simulink model "Model_14Bus_AC_DC_Microgrid"  (R2025a)
settings: Solver=ode23tb  StartTime=0.0  StopTime=0.1  MaxStep=1e-2  RelTol=1e-3
InitFcn:
  | Set_parameters_R2018
StopFcn:
  | Save_Data;
  | Graphics;
undefined symbols (not defined in the file): Clink, D1, Delta, dis1, dis10, dis11, dis12, dis13, dis14, dis2, dis3, dis4, dis5, dis6, dis7, dis8, dis9, Fc, Fnom, Hydride, Increment_MPPT, Ion, Ki_Ireg, Ki_VDCreg, Kp_Ireg, Kp_VDCreg, LimitL_Ireg, LimitL_VDCreg, Limits_MPPT, LimitU_Ireg, LimitU_VDCreg, Lithium, max_min, Metal, Nickel, P_Load_2, P_Load_3, Pnom, Pnom_T1, Pnom_T2, Pnom_T3, Pnom_xfo, Ql_Load_2, Ql_Load_3, R_Load_9, R_Load_DC, RL, Rl, RLff, Rls, sigbuilder_block, Ts, Ts_Control, Ts_Power, V1_LL_T3, Vf, Vfd, Vnom_dc, Vnom_DC, Vnom_Diesel ... (+5)
libraries: spsRMSLib x87, spsCurrentMeasurementLib x47, spsThreePhaseVIMeasurementLib x23, spsVoltageMeasurementLib x21, spsPowerLib x21, spsTHDLib x20, spsThreePhaseSeriesRLCBranchLib x20, spsSeriesRLCBranchLib x19, spsIGBTDiodeLib x14, spsThreePhaseBreakerLib x14, powerlib_extras x14, simulink x12
(part 1 of 9)
settings Model: Creator=Leony  LastModifiedBy=Sanny
settings SolverCC: ZeroCrossAlgorithm=Adaptive  AlgebraicLoopSolver=TrustRegion  SolverResetMethod=Robust
settings DataIOCC: LimitDataPoints=on  SaveFormat=Array  ReturnWorkspaceOutputs=off
settings OptimizationCC: LifeSpan=inf
settings DebuggingCC: AlgebraicLoopMsg=none  UnderspecifiedInitializationDetection=Classic  MergeDetectMultiDrivingBlocksExec=none  IgnoredZcDiagnostic=none  SolverPrmCheckMsg=warning  UnconnectedInputMsg=warning  UnconnectedOutputMsg=warning  UnconnectedLineMsg=warning  AllowSymbolicDim=off  SFUnexpectedBacktrackingDiag=warning  SFNoUnconditionalDefaultTransitionDiag=warning  SFExecutionAtInitializationDiag=none  ArithmeticOperatorsInVariantConditions=warning
settings HardwareCC: ProdBitPerPointer=32.0  ProdBitPerSizeT=32.0  ProdBitPerPtrDiffT=32.0  ProdLargestAtomicFloat=None  ProdIntDivRoundTo=Undefined  ProdEndianess=Unspecified  ProdWordSize=32.0  ProdHWDeviceType=32-bit Generic
settings ModelReferenceCC: EnableRefExpFcnMdlSchedulingChecks=on  PropagateSignalLabelsOutOfModel=off
settings SFSimCC: SimUseLocalCustomCode=off  CustomCodeUndefinedFunction=UseInterfaceOnly
settings RTWCC: RTWUseLocalCustomCode=off  GPUComputeCapability=3.5
settings CodeAppCC: StateflowObjectComments=on
settings GRTTargetCC: TargetLangStandard=C89/C90 (ANSI)
settings ConfigComp: CovMetricSettings=dw  CovSaveCumulativeToWorkspaceVar=on  CovSaveSingleToWorkspaceVar=on  CovExternalEMLEnable=off
settings SimscapeCC: SimscapeNormalizeSystem=off

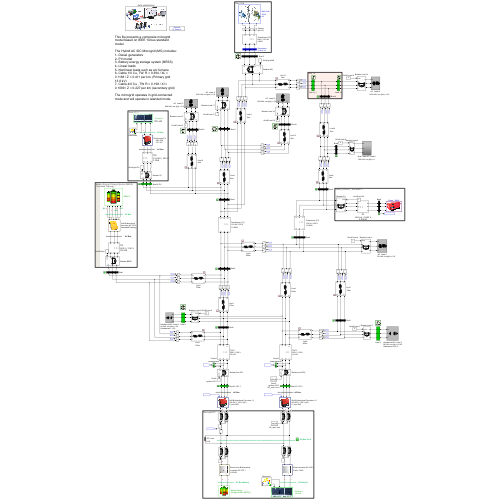
[thumbnail: Simulink's stored preview of the top-level diagram]
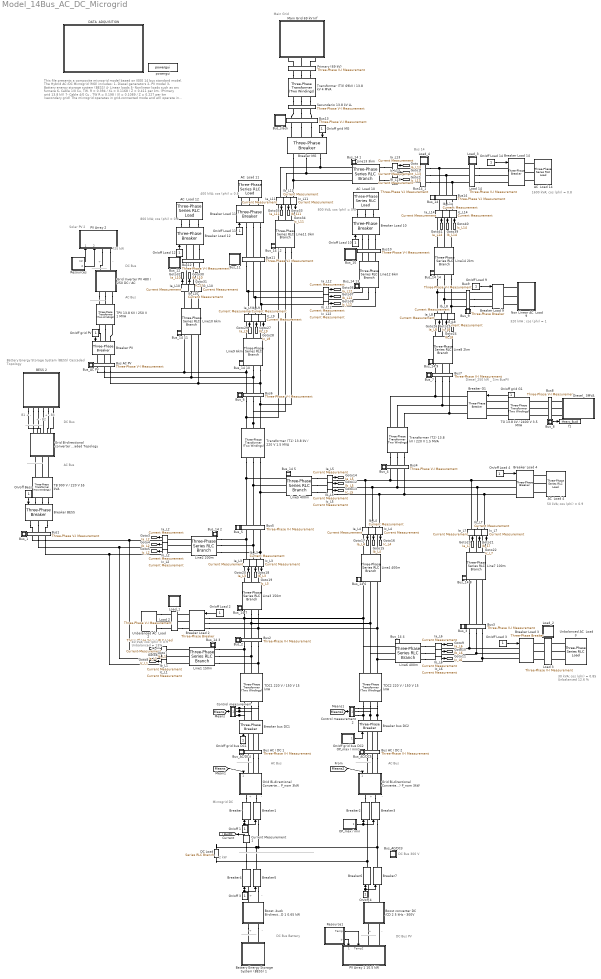
== system Model_14Bus_AC_DC_Microgrid ==
  note: Main Grid
  note: Solar PV 2
  note: Battery Energy Storage System (BESS)
      | Cascaded Topology
  note: ---------------
  note: B1 + -
  note: DC Bus
  note: -
  note: +
  note: This file presents a composite microgrid model based on IEEE 14 bus standard model.
      |
      | The Hybrid AC /DC Microgrid (MG) includes:
      | 1- Diesel generators
      | 2- PV model
      | 3- Battery energy storage system (BESS)
      | 4- Linear loads
      | 5- Nonlinear loads such as arc furnace
      | 6- Cable 1/0 Cu, TW. R = 0.394 / XL = 0.1168 / Z = 0.411 per km. (Primary grid 13.8 kV)
      | 7- Cable 4/0 Cu , TW R = 0.198 / Xl = 0.1089 / Z = 0.227 per km (secondary grid)
      |
      | The microgrid operates in grid-connected mode and will operate in islanded mode.
  note: 725 kW
  note: + - B3
  note: + - B2
  note: DC Bus
  note: AC Bus
  note: AC Bus
  note: ---------------
  note: ---------------
  note: -----------------
  note: 1600 kVA; cos (phi) = 0.8
  note: 800 kVA; cos (phi) = 0.8
  note: 400 kVA; cos (phi) = 0.8
  note: 800 kVA; cos (phi) = 0.8
  note: 50 kVA; cos (phi) = 0.9
  note: 40 kVA; cos (phi) = 0.9
      | Unbalanced = 13%
  note: ---------------
  note: -
  note: ---------------------------------------------------------------------------
  note: AC Bus
  note: +
  note: +
  note: ---------------
  note: DC Bus 300 V
  note: AC Bus
  note: 2 kW
  note: -
  note: Diesel_250 kW _ Sim BusPV
  note: DC Bus Battery
  note: +
  note: -
  note: +
  note: ---------------
  note: -
  note: ---------------
  note: +
  note: -
  note: DC Bus PV
  note: Microgrid DC
  note: 30 kVA; cos (phi) = 0.85
      | Unbalanced 12.6 %
  note: 320 kVA ; cos (phi) = 1
  note: Bus 14
    Ic_L{3..4,7..9,11} (6 alike) : spsCurrentMeasurementLib/Current Measurement  PhasorSimulation=off  OutputType=Complex  PSBequivalent=0
  "  PV Array 1 10.5 kW" : Subsystem
      mask Display: image(imread('Icons\PV.png'));
  "  PV Array 2" : Subsystem
      mask Display: image(imread('Icons\PV.png'));
  " Bus13" : spsThreePhaseVIMeasurementLib/Three-Phase V-I Measurement  VoltageMeasurement=phase-to-ground  SetLabelV=on  LabelV=Vabc_Sec  Vpu=off  VpuLL=off  CurrentMeasurement=yes  SetLabelI=on  LabelI=Iabc_Sec  Ipu=off  Pbase=100e6  Vbase=500e3  OutputType=Complex  PhasorSimulation=off  PSBequivalent=0
  AC  Load 10 : spsThreePhaseSeriesRLCLoadLib/Three-Phase Series RLC Load  LConnTagsString=A|B|C  Configuration=Y (grounded)  NominalVoltage=Vnom_prim  Vabc=[1e3 1e3 1e3]  Vabcp=[1e3 1e3 1e3]  NominalFrequency=Fnom  UnbalancedPower=off  ActivePower=P_Load_10  InductivePower=Ql_Load_10  CapacitivePower=0  Pabc=[10e3 9e3 11e3]  QLabc=[100 90 110]  QCabc=[100 90 110]  Pabcp=[10e3 9e3 11e3]  QLabcp=[100 90 110]  QCabcp=[100 90 110]  Measurements=None  LoadType=constant Z
  AC  Load 11 : spsThreePhaseSeriesRLCLoadLib/Three-Phase Series RLC Load  LConnTagsString=A|B|C  Configuration=Y (grounded)  NominalVoltage=Vnom_prim  Vabc=[1e3 1e3 1e3]  Vabcp=[1e3 1e3 1e3]  NominalFrequency=Fnom  UnbalancedPower=off  ActivePower=P_Load_11  InductivePower=Ql_Load_11  CapacitivePower=0  Pabc=[10e3 9e3 11e3]  QLabc=[100 90 110]  QCabc=[100 90 110]  Pabcp=[10e3 9e3 11e3]  QLabcp=[100 90 110]  QCabcp=[100 90 110]  Measurements=None  LoadType=constant Z
  AC  Load 12 : spsThreePhaseSeriesRLCLoadLib/Three-Phase Series RLC Load  LConnTagsString=A|B|C  Configuration=Y (grounded)  NominalVoltage=Vnom_prim  Vabc=[1e3 1e3 1e3]  Vabcp=[1e3 1e3 1e3]  NominalFrequency=Fnom  UnbalancedPower=off  ActivePower=P_Load_12  InductivePower=Ql_Load_12  CapacitivePower=0  Pabc=[10e3 9e3 11e3]  QLabc=[100 90 110]  QCabc=[100 90 110]  Pabcp=[10e3 9e3 11e3]  QLabcp=[100 90 110]  QCabcp=[100 90 110]  Measurements=None  LoadType=constant Z
  AC  Load 14 : spsThreePhaseSeriesRLCLoadLib/Three-Phase Series RLC Load  LConnTagsString=A|B|C  Configuration=Y (grounded)  NominalVoltage=Vnom_prim  Vabc=[1e3 1e3 1e3]  Vabcp=[1e3 1e3 1e3]  NominalFrequency=Fnom  UnbalancedPower=off  ActivePower=P_Load_14  InductivePower=Ql_Load_14  CapacitivePower=0  Pabc=[10e3 9e3 11e3]  QLabc=[100 90 110]  QCabc=[100 90 110]  Pabcp=[10e3 9e3 11e3]  QLabcp=[100 90 110]  QCabcp=[100 90 110]  Measurements=None  LoadType=constant Z
  AC  Load 4 : spsThreePhaseSeriesRLCLoadLib/Three-Phase Series RLC Load  LConnTagsString=A|B|C  Configuration=Y (grounded)  NominalVoltage=Vnom_sec  Vabc=[1e3 1e3 1e3]  Vabcp=[1e3 1e3 1e3]  NominalFrequency=Fnom  UnbalancedPower=off  ActivePower=P_Load_4  InductivePower=Ql_Load_4  CapacitivePower=0  Pabc=[10e3 9e3 11e3]  QLabc=[100 90 110]  QCabc=[100 90 110]  Pabcp=[10e3 9e3 11e3]  QLabcp=[100 90 110]  QCabcp=[100 90 110]  Measurements=None  LoadType=constant Z
  "BESS 2 " : Subsystem
      mask Display: image('Icons\Battery Energy Storage System (BESS).png');
  Battery Energy Storage System (BESS) 1 : Subsystem
      mask Display: image('Icons\Battery Energy Storage System (BESS).png');
  Boost -buck Bi-directional converter DC /CD 1 0.65 kW : Subsystem
      mask Display: image(imread('Icons\DC_DC_Converter.jpg'));
  "Boost converter DC /CD 2 5 kHz - 300V " : Subsystem
      mask Display: image(imread('Icons\DC_DC_Converter.jpg'));
  Breaker{,1..7} (8 alike) : spsBreakerLib/Breaker  InitialState=1  SwitchingTimes="[1/60  5/60]"  External=on  BreakerResistance=0.01  SnubberResistance=1e6  SnubberCapacitance=inf  Measurements=None  MoreParameters=on  NoBreakLoop=off
  "Breaker BESS " : spsThreePhaseBreakerLib/Three-Phase Breaker  InitialState=closed  SwitchA=on  SwitchB=on  SwitchC=on  SwitchTimes="[4/60  10/60]"  External=on  BreakerResistance=0.001  SnubberResistance=1e6  SnubberCapacitance=inf  Measurements=None
  Breaker G1 : spsThreePhaseBreakerLib/Three-Phase Breaker  InitialState=closed  SwitchA=on  SwitchB=on  SwitchC=on  SwitchTimes="[4/60  10/60]"  External=on  BreakerResistance=0.001  SnubberResistance=1e6  SnubberCapacitance=inf  Measurements=None
  Breaker Load {2..4,9..12,14} (8 alike) : spsThreePhaseBreakerLib/Three-Phase Breaker  InitialState=closed  SwitchA=on  SwitchB=on  SwitchC=on  SwitchTimes="[4/60  10/60]"  External=on  BreakerResistance=0.001  SnubberResistance=1e6  SnubberCapacitance=inf  Measurements=None
  Breaker MG : spsThreePhaseBreakerLib/Three-Phase Breaker  InitialState=closed  SwitchA=on  SwitchB=on  SwitchC=on  SwitchTimes="[4/60  10/60]"  External=on  BreakerResistance=0.001  SnubberResistance=1e6  SnubberCapacitance=inf  Measurements=None
  Breaker PV : spsThreePhaseBreakerLib/Three-Phase Breaker  InitialState=closed  SwitchA=on  SwitchB=on  SwitchC=on  SwitchTimes="[4/60  10/60]"  External=on  BreakerResistance=0.001  SnubberResistance=1e6  SnubberCapacitance=inf  Measurements=None
  Breaker bus DC1 : spsThreePhaseBreakerLib/Three-Phase Breaker  InitialState=closed  SwitchA=on  SwitchB=on  SwitchC=on  SwitchTimes="[4/60  10/60]"  External=on  BreakerResistance=0.001  SnubberResistance=1e6  SnubberCapacitance=inf  Measurements=None
  Breaker bus DC2 : spsThreePhaseBreakerLib/Three-Phase Breaker  InitialState=closed  SwitchA=on  SwitchB=on  SwitchC=on  SwitchTimes="[4/60  10/60]"  External=on  BreakerResistance=0.001  SnubberResistance=1e6  SnubberCapacitance=inf  Measurements=None
  Bus AC / DC 1 : spsThreePhaseVIMeasurementLib/Three-Phase V-I Measurement  VoltageMeasurement=phase-to-ground  SetLabelV=on  LabelV=Vabc_B1_busDC1  Vpu=off  VpuLL=off  CurrentMeasurement=yes  SetLabelI=on  LabelI=Iabc_B1_busDC1  Ipu=off  Pbase=100e6  Vbase=25e3  OutputType=Complex  PhasorSimulation=off  PSBequivalent=0
  Bus AC / DC 2 : spsThreePhaseVIMeasurementLib/Three-Phase V-I Measurement  VoltageMeasurement=phase-to-ground  SetLabelV=on  LabelV=Vabc_B1_busDC2  Vpu=off  VpuLL=off  CurrentMeasurement=yes  SetLabelI=on  LabelI=Iabc_B1_busDC2  Ipu=off  Pbase=100e6  Vbase=25e3  OutputType=Complex  PhasorSimulation=off  PSBequivalent=0
  Bus AC PV : spsThreePhaseVIMeasurementLib/Three-Phase V-I Measurement  VoltageMeasurement=phase-to-ground  SetLabelV=on  LabelV=Vabc_B1  Vpu=off  VpuLL=off  CurrentMeasurement=yes  SetLabelI=on  LabelI=Iabc_B1  Ipu=off  Pbase=100e6  Vbase=25e3  OutputType=Complex  PhasorSimulation=off  PSBequivalent=0
  Bus1 : spsThreePhaseVIMeasurementLib/Three-Phase V-I Measurement  VoltageMeasurement=phase-to-ground  SetLabelV=on  LabelV=VabcLL_Bus_1  Vpu=off  VpuLL=off  CurrentMeasurement=yes  SetLabelI=on  LabelI=IabcLL_Bus_1  Ipu=off  Pbase=100e6  Vbase=380/sqrt(2)  OutputType=Complex  PhasorSimulation=off  PSBequivalent=0
  Bus10 : spsThreePhaseVIMeasurementLib/Three-Phase V-I Measurement  VoltageMeasurement=phase-to-ground  SetLabelV=on  LabelV=VabcLL_Bus_10  Vpu=off  VpuLL=off  CurrentMeasurement=yes  SetLabelI=on  LabelI=IabcLL_Bus_10  Ipu=off  Pbase=100e6  Vbase=25e3/sqrt(2)  OutputType=Complex  PhasorSimulation=off  PSBequivalent=0
  Bus11 : spsThreePhaseVIMeasurementLib/Three-Phase V-I Measurement  VoltageMeasurement=phase-to-ground  SetLabelV=on  LabelV=VabcLL_Bus_11  Vpu=off  VpuLL=off  CurrentMeasurement=yes  SetLabelI=on  LabelI=IabcLL_Bus_11  Ipu=off  Pbase=100e6  Vbase=25e3/sqrt(2)  OutputType=Complex  PhasorSimulation=off  PSBequivalent=0
  Bus12 : spsThreePhaseVIMeasurementLib/Three-Phase V-I Measurement  VoltageMeasurement=phase-to-ground  SetLabelV=on  LabelV=VabcLL_Bus_12  Vpu=off  VpuLL=off  CurrentMeasurement=yes  SetLabelI=on  LabelI=IabcLL_Bus_12  Ipu=off  Pbase=100e6  Vbase=25e3  OutputType=Complex  PhasorSimulation=off  PSBequivalent=0
  Bus14 : spsThreePhaseVIMeasurementLib/Three-Phase V-I Measurement  VoltageMeasurement=phase-to-ground  SetLabelV=on  LabelV=VabcLL_Bus_14  Vpu=off  VpuLL=off  CurrentMeasurement=yes  SetLabelI=on  LabelI=IabcLL_Bus_14  Ipu=off  Pbase=100e6  Vbase=25e3/sqrt(2)  OutputType=Complex  PhasorSimulation=off  PSBequivalent=0
  Bus14_1 : spsThreePhaseVIMeasurementLib/Three-Phase V-I Measurement  VoltageMeasurement=phase-to-ground  SetLabelV=on  LabelV=Vabc_load_14_1  Vpu=off  VpuLL=off  CurrentMeasurement=yes  SetLabelI=on  LabelI=Iabc_load_14_1  Ipu=off  Pbase=100e6  Vbase=380/sqrt(2)  OutputType=Complex  PhasorSimulation=off  PSBequivalent=0
  Bus2 : spsThreePhaseVIMeasurementLib/Three-Phase V-I Measurement  VoltageMeasurement=phase-to-ground  SetLabelV=on  LabelV=VabcLL_Bus_2  Vpu=off  VpuLL=off  CurrentMeasurement=yes  SetLabelI=on  LabelI=IabcLL_Bus_2  Ipu=off  Pbase=100e6  Vbase=380/sqrt(2)  OutputType=Complex  PhasorSimulation=off  PSBequivalent=0
  Bus3 : spsThreePhaseVIMeasurementLib/Three-Phase V-I Measurement  VoltageMeasurement=phase-to-ground  SetLabelV=on  LabelV=VabcLL_Bus_3  Vpu=off  VpuLL=off  CurrentMeasurement=yes  SetLabelI=on  LabelI=IabcLL_Bus_3  Ipu=off  Pbase=100e6  Vbase=500e3  OutputType=Complex  PhasorSimulation=off  PSBequivalent=0
  Bus4 : spsThreePhaseVIMeasurementLib/Three-Phase V-I Measurement  VoltageMeasurement=phase-to-ground  SetLabelV=on  LabelV=VabcLL_Bus_4  Vpu=off  VpuLL=off  CurrentMeasurement=yes  SetLabelI=on  LabelI=IabcLL_Bus_4  Ipu=off  Pbase=100e6  Vbase=380/sqrt(2)  OutputType=Complex  PhasorSimulation=off  PSBequivalent=0
  Bus5 : spsThreePhaseVIMeasurementLib/Three-Phase V-I Measurement  VoltageMeasurement=phase-to-ground  SetLabelV=on  LabelV=VabcLL_Bus_5  Vpu=off  VpuLL=off  CurrentMeasurement=yes  SetLabelI=on  LabelI=IabcLL_Bus_5  Ipu=off  Pbase=100e6  Vbase=380/sqrt(2)  OutputType=Complex  PhasorSimulation=off  PSBequivalent=0
  Bus6 : spsThreePhaseVIMeasurementLib/Three-Phase V-I Measurement  VoltageMeasurement=phase-to-ground  SetLabelV=on  LabelV=VabcLL_Bus_6  Vpu=off  VpuLL=off  CurrentMeasurement=yes  SetLabelI=on  LabelI=IabcLL_Bus_6  Ipu=off  Pbase=100e6  Vbase=25e3/sqrt (2)  OutputType=Complex  PhasorSimulation=off  PSBequivalent=0
  Bus7 : spsThreePhaseVIMeasurementLib/Three-Phase V-I Measurement  VoltageMeasurement=phase-to-ground  SetLabelV=on  LabelV=VabcLL_Bus_7  Vpu=off  VpuLL=off  CurrentMeasurement=yes  SetLabelI=on  LabelI=IabcLL_Bus_7  Ipu=off  Pbase=100e6  Vbase=25e3/sqrt(2)  OutputType=Complex  PhasorSimulation=off  PSBequivalent=0
  Bus8 : spsThreePhaseVIMeasurementLib/Three-Phase V-I Measurement  VoltageMeasurement=phase-to-ground  SetLabelV=on  LabelV=VabcLL_Bus_8  Vpu=off  VpuLL=off  CurrentMeasurement=yes  SetLabelI=on  LabelI=IabcLL_Bus_8  Ipu=off  Pbase=100e6  Vbase=25e3/sqrt(2)  OutputType=Complex  PhasorSimulation=off  PSBequivalent=0
  Bus9 : spsThreePhaseVIMeasurementLib/Three-Phase V-I Measurement  VoltageMeasurement=phase-to-ground  SetLabelV=on  LabelV=VabcLL_Bus_9  Vpu=off  VpuLL=off  CurrentMeasurement=yes  SetLabelI=on  LabelI=IabcLL_Bus_9  Ipu=off  Pbase=100e6  Vbase=25e3/sqrt(2)  OutputType=Complex  PhasorSimulation=off  PSBequivalent=0
  Bus_1 : Subsystem
  Bus_10 : Subsystem
      mask Display: image('Icons\S_meeter.png');
  Bus_11 : Subsystem
      mask Display: image('Icons\S_meeter.png');
  Bus_12 : Subsystem
      mask Display: image('Icons\S_meeter.png');
  "Bus_14 " : Subsystem
  Bus_14 1 : Subsystem
  Bus_14 10 : Subsystem
  Bus_14 11 : Subsystem
  Bus_14 12 : Subsystem
  Bus_14 13 : Subsystem
  Bus_14 14 : Subsystem
  Bus_14 2 : Subsystem
  Bus_14 3 : Subsystem
  Bus_14 4 : Subsystem
  Bus_14 5 : Subsystem
  Bus_14 6 : Subsystem
  Bus_14 7 : Subsystem
  Bus_14 8 : Subsystem
  Bus_14 9 : Subsystem
  Bus_2 : Subsystem
  Bus_3 : Subsystem
  Bus_4 : Subsystem
  Bus_5 : Subsystem
  "Bus_6 " : Subsystem
  Bus_7 : Subsystem
  "Bus_8      " : Subsystem
  Bus_9 : Subsystem
  "Bus_AC PV " : Subsystem
  Bus_AC/DC3 : Subsystem
  Bus_AC/DC4 : Subsystem
  Bus_AC/DC5 : Subsystem
  "Bus_slack " : Subsystem
      mask Display: image('Icons\S_meeter.png');
  Control measurement : Subsystem
  Control measurement2 : Subsystem
  Current Measurement1 : spsCurrentMeasurementLib/Current Measurement  PhasorSimulation=off  OutputType=Complex  PSBequivalent=0
  DATA  ADQUISITION : Subsystem
      mask Display: image('Icons\SCADA.png');
  DC Load : spsSeriesRLCBranchLib/Series RLC Branch  LConnTagsString=__new0  RConnTagsString=__new0  BranchType=R  Resistance=R_Load_DC  Inductance=1e-3  SetiL0=off  InitialCurrent=0  Capacitance=1e-6  Setx0=off  InitialVoltage=0  Measurements=None
  Diesel_ 3MVA : Subsystem
      mask Display: image(imread('Icons\Diesel 50kW1.png'));
  Grid Bi-directional converter AC /CD 2 Cascaded Topology : Subsystem
      mask Display: image(imread('Icons\Bi-directional converter.png'));
  Grid Bi-directional Converter 1.1 300 (DC) / 150 V (AC) P_nom 3kW : Subsystem
      mask Display: image(imread('Icons\Inverter.png'));
  Grid Bi-directional Converter 1.2 300 (DC) / 150 V (AC) P_nom 3kW : Subsystem
      mask Display: image(imread('Icons\Inverter.png'));
  "Grid Inverter PV 480 / 250 DC / AC " : Subsystem
      mask Display: image(imread('Icons\Inverter.png'));
  Ia_L{1..14} (14 alike) : spsCurrentMeasurementLib/Current Measurement  PhasorSimulation=off  OutputType=Complex  PSBequivalent=0
  Ib_L{1..14} (14 alike) : spsCurrentMeasurementLib/Current Measurement  PhasorSimulation=off  OutputType=Complex  PSBequivalent=0
  Ic_L{1..2,5..6,10,12..14} (8 alike) : spsCurrentMeasurementLib/Current Measurement  PhasorSimulation=off  OutputType=Complex  PSBequivalent=0
  Line1 150m : spsThreePhaseSeriesRLCBranchLib/Three-Phase Series RLC Branch  LConnTagsString=A|B|C  RConnTagsString=A|B|C  BranchType=RL  Resistance=Rls * dis1  Inductance=Xls / 377 * dis1  Capacitance=1e-6  Measurements=None
  Line10 6km : spsThreePhaseSeriesRLCBranchLib/Three-Phase Series RLC Branch  LConnTagsString=A|B|C  RConnTagsString=A|B|C  BranchType=RL  Resistance=Rl * dis10  Inductance=Xl/377 * dis10  Capacitance=1e-6  Measurements=None
  Line11 3km : spsThreePhaseSeriesRLCBranchLib/Three-Phase Series RLC Branch  LConnTagsString=A|B|C  RConnTagsString=A|B|C  BranchType=RL  Resistance=Rl* dis11  Inductance=Xl/377 * dis11  Capacitance=1e-6  Measurements=None
  Line12 6km : spsThreePhaseSeriesRLCBranchLib/Three-Phase Series RLC Branch  LConnTagsString=A|B|C  RConnTagsString=A|B|C  BranchType=RL  Resistance=Rl * dis12  Inductance=Xl/377 * dis12  Capacitance=1e-6  Measurements=None
  Line13 3km : spsThreePhaseSeriesRLCBranchLib/Three-Phase Series RLC Branch  LConnTagsString=A|B|C  RConnTagsString=A|B|C  BranchType=RL  Resistance=Rl * dis13  Inductance=Xl/377 * dis13  Capacitance=1e-6  Measurements=None
  Line14 2km : spsThreePhaseSeriesRLCBranchLib/Three-Phase Series RLC Branch  LConnTagsString=A|B|C  RConnTagsString=A|B|C  BranchType=RL  Resistance=Rl * dis14  Inductance=Xl/377 * dis14  Capacitance=1e-6  Measurements=None
  Line2 200m : spsThreePhaseSeriesRLCBranchLib/Three-Phase Series RLC Branch  LConnTagsString=A|B|C  RConnTagsString=A|B|C  BranchType=RL  Resistance=Rls * dis2  Inductance=Xls/377 * dis2  Capacitance=1e-6  Measurements=None
  Line3 150m : spsThreePhaseSeriesRLCBranchLib/Three-Phase Series RLC Branch  LConnTagsString=A|B|C  RConnTagsString=A|B|C  BranchType=RL  Resistance=Rls * dis3  Inductance=Xls/377 * dis3  Capacitance=1e-6  Measurements=None
  Line4 400m : spsThreePhaseSeriesRLCBranchLib/Three-Phase Series RLC Branch  LConnTagsString=A|B|C  RConnTagsString=A|B|C  BranchType=RL  Resistance=Rls * dis4  Inductance=Xls/377 * dis4  Capacitance=1e-6  Measurements=None
  Line5 400m : spsThreePhaseSeriesRLCBranchLib/Three-Phase Series RLC Branch  LConnTagsString=A|B|C  RConnTagsString=A|B|C  BranchType=RL  Resistance=Rls * dis5  Inductance=Xls/377 * dis5  Capacitance=1e-6  Measurements=None
  Line6 400m : spsThreePhaseSeriesRLCBranchLib/Three-Phase Series RLC Branch  LConnTagsString=A|B|C  RConnTagsString=A|B|C  BranchType=RL  Resistance=Rls * dis6  Inductance=Xls/377 * dis6  Capacitance=1e-6  Measurements=None
  Line7 100m : spsThreePhaseSeriesRLCBranchLib/Three-Phase Series RLC Branch  LConnTagsString=A|B|C  RConnTagsString=A|B|C  BranchType=RL  Resistance=Rls * dis7  Inductance=Xls/377 * dis7  Capacitance=1e-6  Measurements=None
  Line8 2km : spsThreePhaseSeriesRLCBranchLib/Three-Phase Series RLC Branch  LConnTagsString=A|B|C  RConnTagsString=A|B|C  BranchType=RL  Resistance=Rl * dis8  Inductance=Xl/377 * dis8  Capacitance=1e-6  Measurements=None
  Line9 6km : spsThreePhaseSeriesRLCBranchLib/Three-Phase Series RLC Branch  LConnTagsString=A|B|C  RConnTagsString=A|B|C  BranchType=RL  Resistance=Rl * dis9  Inductance=Xl/377 * dis9  Capacitance=1e-6  Measurements=None
  Load 14 : spsThreePhaseVIMeasurementLib/Three-Phase V-I Measurement  VoltageMeasurement=phase-to-ground  SetLabelV=on  LabelV=Vabc_load_14  Vpu=off  VpuLL=off  CurrentMeasurement=yes  SetLabelI=on  LabelI=Iabc_load_14  Ipu=off  Pbase=100e6  Vbase=380/sqrt(2)  OutputType=Complex  PhasorSimulation=off  PSBequivalent=0
  Load 2 : spsThreePhaseVIMeasurementLib/Three-Phase V-I Measurement  VoltageMeasurement=phase-to-ground  SetLabelV=on  LabelV=Vabc_load_1  Vpu=off  VpuLL=off  CurrentMeasurement=yes  SetLabelI=on  LabelI=Iabc_load_1  Ipu=off  Pbase=100e6  Vbase=380/sqrt(2)  OutputType=Complex  PhasorSimulation=off  PSBequivalent=0
  Load 3 : spsThreePhaseVIMeasurementLib/Three-Phase V-I Measurement  VoltageMeasurement=phase-to-ground  SetLabelV=on  LabelV=Vabc_load_2  Vpu=off  VpuLL=off  CurrentMeasurement=yes  SetLabelI=on  LabelI=Iabc_load_2  Ipu=off  Pbase=100e6  Vbase=380/sqrt(2)  OutputType=Complex  PhasorSimulation=off  PSBequivalent=0
  Load_1 : Subsystem
      mask Display: image('Icons\S_meeter.png');
  Load_2 : Subsystem
      mask Display: image('Icons\S_meeter.png');
  Load_3 : Subsystem
      mask Display: image('Icons\S_meeter.png');
  Load_4 : Subsystem
      mask Display: image('Icons\S_meeter.png');
  Main Grid 69 kV Inf : Subsystem
      mask Display: image('Icons\Main-grid.png');
  Non Linear AC  Load 9 : Subsystem
  OP_max / min : Subsystem
  On/off grid bus DC1 : Constant
  On/off grid bus DC2 OP_max / min1 : Subsystem
  On/off 1 : Constant
  On/off 3 : Constant
  On/off 4 : Constant
  On/off Bess : Constant
  On/off Load {2..4,9..12,14} (8 alike) : Constant
  On/off grid G1 : Constant
  On/off grid MG : Constant
  On/off grid PV : Constant
  Primary (69 kV) : spsThreePhaseVIMeasurementLib/Three-Phase V-I Measurement  VoltageMeasurement=phase-to-ground  SetLabelV=on  LabelV=Vabc_Prim_pu  Vpu=off  VpuLL=on  CurrentMeasurement=yes  SetLabelI=on  LabelI=Iabc_Prim  Ipu=on  Pbase=100e6  Vbase=69e3/sqrt(2)  OutputType=Magnitude  PhasorSimulation=off  PSBequivalent=0
  Resource1 : Subsystem
      mask Display: image(imread('Icons\R_Sol.jpg'));
  Resources : Subsystem
      mask Display: image(imread('Icons\R_Sol.jpg'));
  Secundario 13.8 kV LL : spsThreePhaseVIMeasurementLib/Three-Phase V-I Measurement  VoltageMeasurement=phase-to-phase  SetLabelV=on  LabelV=Vabc_Sec_pu  Vpu=off  VpuLL=on  CurrentMeasurement=yes  SetLabelI=on  LabelI=Iabc_Sec_pu  Ipu=off  Pbase=250e6  Vbase=Vnom_prim/sqrt(2)  OutputType=Magnitude  PhasorSimulation=off  PSBequivalent=0
  TB 900 V / 220 V 55 kVA : spsThreePhaseTransformerTwoWindingsLib/Three-Phase Transformer (Two Windings)  Winding1Connection=Delta (D1)  Winding2Connection=Y  CoreType=Three single-phase transformers  SetSaturation=off  Hysteresis=off  DataFile='hysteresis'  SetInitialFlux=off  Measurements=None  UNITS=pu  NominalPower=[ 55e3 , Fnom ]  Winding1=[ 900 , 0.0015 , 0.03]  Winding2=[ Vnom_sec , 0.0015 , 0.03 ]  Rm=200  Lm=200  L0=0.5  Saturation="[ 0,0  ;  0.005,1.2  ;  1.0,1.4 ]"  InitialFluxes=[ 0.8 , -0.8 , 0.7 ]  BreakLoop=off  DiscreteSolver=Trapezoidal iterative  DataType=off  TransfoNumber=0
  TDC1 220 V / 150 V 15 kVA : spsThreePhaseTransformerTwoWindingsLib/Three-Phase Transformer (Two Windings)  Winding1Connection=Y  Winding2Connection=Y  CoreType=Three single-phase transformers  SetSaturation=off  Hysteresis=off  DataFile='hysteresis'  SetInitialFlux=off  Measurements=None  UNITS=pu  NominalPower=[15e3 , Fnom ]  Winding1=[Vnom_sec , 0.03/2 , 0.03/377]  Winding2=[Vnom_ter_AC_DC , 0.03/2 , 0.03/377]  Rm=500  Lm=500  L0=0.5  Saturation=[ 0,0 ; 0.0024,1.2 ; 1.0,1.52 ]  InitialFluxes=[ 0.8 , -0.8 , 0.7 ]  BreakLoop=off  DiscreteSolver=Trapezoidal iterative  DataType=off  TransfoNumber=1
  TDC2 220 V / 150 V 15 kVA : spsThreePhaseTransformerTwoWindingsLib/Three-Phase Transformer (Two Windings)  Winding1Connection=Y  Winding2Connection=Y  CoreType=Three single-phase transformers  SetSaturation=off  Hysteresis=off  DataFile='hysteresis'  SetInitialFlux=off  Measurements=None  UNITS=pu  NominalPower=[15e3 , Fnom ]  Winding1=[Vnom_sec , 0.03/2 , 0.03/377 ]  Winding2=[Vnom_ter_AC_DC , 0.03/2 , 0.03/377 ]  Rm=500  Lm=500  L0=0.5  Saturation=[ 0,0 ; 0.0024,1.2 ; 1.0,1.52 ]  InitialFluxes=[ 0.8 , -0.8 , 0.7 ]  BreakLoop=off  DiscreteSolver=Trapezoidal iterative  DataType=off  TransfoNumber=1
  TG 13.8 kV / 2400 V 3.5 MVA : spsThreePhaseTransformerTwoWindingsLib/Three-Phase Transformer (Two Windings)  Winding1Connection=Yg  Winding2Connection=Delta (D1)  CoreType=Three single-phase transformers  SetSaturation=off  Hysteresis=off  DataFile='hysteresis'  SetInitialFlux=off  Measurements=None  UNITS=pu  NominalPower=[3.5e6 , Fnom ]  Winding1=[ Vnom_prim , 0.015/2 , 0.015/2/377]  Winding2=[ Vnom_Diesel , 0.015/2 , 0.015/2/377]  Rm=500  Lm=500  L0=0.5  Saturation="[ 0,0  ;  0.005,1.2  ;  1.0,1.4 ]"  InitialFluxes=[ 0.8 , -0.8 , 0.7 ]  BreakLoop=off  DiscreteSolver=Trapezoidal iterative  DataType=off  TransfoNumber=0
  TPV 13.8 KV / 250 V 1 MVA : spsThreePhaseTransformerTwoWindingsLib/Three-Phase Transformer (Two Windings)  Winding1Connection=Yg  Winding2Connection=Delta (D1)  CoreType=Three single-phase transformers  SetSaturation=off  Hysteresis=off  DataFile='hysteresis'  SetInitialFlux=off  Measurements=None  UNITS=pu  NominalPower=[Pnom_xfo, Fnom ]  Winding1=W1_xfo  Winding2=W2_xfo  Rm=Rm_xfo  Lm=Lm_xfo  L0=0.5  Saturation=[ 0,0 ; 0.0024,1.2 ; 1.0,1.52 ]  InitialFluxes=[ 0.8 , -0.8 , 0.7 ]  BreakLoop=off  DiscreteSolver=Trapezoidal iterative  DataType=off  TransfoNumber=0
  Transformer (T1) 13.8 kV / 220 V 1.5 MVA : spsThreePhaseTransformerTwoWindingsLib/Three-Phase Transformer (Two Windings)  Winding1Connection=Y  Winding2Connection=Y  CoreType=Three single-phase transformers  SetSaturation=off  Hysteresis=off  DataFile='hysteresis'  SetInitialFlux=off  Measurements=None  UNITS=pu  NominalPower=[ Pnom_T1, Fnom ]  Winding1=[Vnom_prim , 0.03/2 , 0.03/(2*377) ]  Winding2=[Vnom_sec , 0.03/2 , 0.03/(2*377) ]  Rm=500  Lm=500  L0=0.5  Saturation=[ 0,0 ; 0.0024,1.2 ; 1.0,1.52 ]  InitialFluxes=[ 0.8 , -0.8 , 0.7 ]  BreakLoop=off  DiscreteSolver=Trapezoidal iterative  DataType=off  TransfoNumber=1
  Transformer (T2) 13.8 kV / 220 V 1.5 MVA : spsThreePhaseTransformerTwoWindingsLib/Three-Phase Transformer (Two Windings)  Winding1Connection=Y  Winding2Connection=Y  CoreType=Three single-phase transformers  SetSaturation=off  Hysteresis=off  DataFile='hysteresis'  SetInitialFlux=off  Measurements=None  UNITS=pu  NominalPower=[Pnom_T2 , Fnom]  Winding1=[ Vnom_prim, 0.03/2 , 0.03/(2*377) ]  Winding2=[Vnom_sec , 0.03/2 , 0.03/(2*377) ]  Rm=500  Lm=500  L0=0.5  Saturation=[ 0,0 ; 0.0024,1.2 ; 1.0,1.52 ]  InitialFluxes=[ 0.8 , -0.8 , 0.7 ]  BreakLoop=off  DiscreteSolver=Trapezoidal iterative  DataType=off  TransfoNumber=1
  Transformer (T3) 69kV / 13.8 kV 4 MVA : spsThreePhaseTransformerTwoWindingsLib/Three-Phase Transformer (Two Windings)  Winding1Connection=Yg  Winding2Connection=Delta (D1)  CoreType=Three single-phase transformers  SetSaturation=off  Hysteresis=off  DataFile='hysteresis'  SetInitialFlux=off  Measurements=None  UNITS=pu  NominalPower=[Pnom_T3 , Fnom ]  Winding1=[V1_LL_T3 , 0.015/2 , 0.015/(2*377)]  Winding2=[ Vnom_prim, 0.015/2 , 0.015/(2*377)]  Rm=500  Lm=500  L0=0.5  Saturation="[ 0,0  ;  0.005,1.2  ;  1.0,1.4 ]"  InitialFluxes=[ 0.8 , -0.8 , 0.7 ]  BreakLoop=off  DiscreteSolver=Trapezoidal iterative  DataType=off  TransfoNumber=0
  Unbalanced AC  Load 2 : spsThreePhaseSeriesRLCLoadLib/Three-Phase Series RLC Load  LConnTagsString=A|B|C  Configuration=Y (grounded)  NominalVoltage=Vnom_sec  Vabc=[Vnom_sec/sqrt(3), Vnom_sec/sqrt(3), Vnom_sec/sqrt(3)]  Vabcp=[1e3 1e3 1e3]  NominalFrequency=Fnom  UnbalancedPower=on  ActivePower=P_Load_2  InductivePower=Ql_Load_2  CapacitivePower=0  Pabc=[P_Load_2, P_Load_2*0.85, P_Load_2*1.05]  QLabc=[Ql_Load_2, Ql_Load_2*0.85, Ql_Load_2*1.05]  QCabc=[0 0 0]  Pabcp=[10e3 9e3 11e3]  QLabcp=[100 90 110]  QCabcp=[100 90 110]  Measurements=None  LoadType=constant PQ
  Unbalanced AC  Load 3 : spsThreePhaseSeriesRLCLoadLib/Three-Phase Series RLC Load  LConnTagsString=A|B|C  Configuration=Y (grounded)  NominalVoltage=Vnom_sec  Vabc=[Vnom_sec/sqrt(3), Vnom_sec/sqrt(3), Vnom_sec/sqrt(3)]  Vabcp=[1e3 1e3 1e3]  NominalFrequency=Fnom  UnbalancedPower=on  ActivePower=P_Load_3  InductivePower=Ql_Load_3  CapacitivePower=0  Pabc=[P_Load_3*1.04, P_Load_3, P_Load_3*0.9]  QLabc=[Ql_Load_3*1.04, Ql_Load_3, Ql_Load_3*0.9]  QCabc=[0 0 0]  Pabcp=[10e3 9e3 11e3]  QLabcp=[100 90 110]  QCabcp=[100 90 110]  Measurements=None  LoadType=constant Z
  f1 : ToWorkspace  VariableName=Means_Bus8  SaveFormat=Timeseries  SampleTime=-1
  powergui : spspowerguiLib/powergui  Priority=1  SimulationMode=Discrete  SampleTime=Ts_Power  frequency=60  Iterations=50  frequencyindice=60  Pbase=100e6  ErrMax=1e-4  UnitsV=kV  UnitsW=MW  buscounter=0  FunctionMessages=off  echomessages=off  EnableUseOfTLC=off  CurrentSourceSwitches=off  DisableSnubberDevices=off  DisableRonSwitches=off  DisableVfSwitches=off  DisplayEquations=off  AutomaticDiscreteSolvers=off  SolverType=Tustin  Interpol=off  ExternalGateDelay=off  methode=off  Ts=0  x0status=blocks  SPID=off  SwTol=0  HookPort=off  NonlinearTolerance=1e-4  nMaxIteration=100  ContinueOnMaxIteration=off  RestoreLinks=warning  ResistiveCurrentMeasurement=off  Frange=[0:2:500]  Ylog=off  Xlog=on  ShowGrid=off  save=off  variable=ZData  structure=0  ZoomFFT=off  StartTime=0.0  cycles=1  DisplayStyle=1  fundamental=60  FreqAxis=off  MaxFrequency=1000  frequencyindicesteady=1  RmsSteady=1  display=off
  tag scope: I_BusDC=global, Ia_L10=global, Ia_L11=global, Ia_L12=global, Ia_L13=global, Ia_L14=global, Ia_L1=global, Ia_L2=global, Ia_L3=global, Ia_L4=global, Ia_L5=global, Ia_L6=global, Ia_L7=global, Ia_L8=global, Ia_L9=global, Ib_L10=global, Ib_L11=global, Ib_L12=global, Ib_L13=global, Ib_L14=global, Ib_L1=global, Ib_L2=global, Ib_L3=global, Ib_L4=global, Ib_L5=global, Ib_L6=global, Ib_L7=global, Ib_L8=global, Ib_L9=global, Ic_L10=global, Ic_L11=global, Ic_L12=global, Ic_L13=global, Ic_L14=global, Ic_L1=global, Ic_L2=global, Ic_L3=global, Ic_L4=global, Ic_L5=global, Ic_L6=global, Ic_L7=global, Ic_L8=global, Ic_L9=global, Means2=global, Means=global
  wires:
  On/off grid PV/1 -> Breaker PV/1
  On/off Bess/1 -> "Breaker BESS "/1
  On/off grid MG/1 -> Breaker MG/1
  Ia_L13/1 -> [Ia_L13]
  Ib_L13/1 -> [Ib_L13]
  Ic_L13/1 -> [Ic_L13]
  Resources/1(Ir2) -> "  PV Array 2"/1(Irradiance)
  On/off Load 12/1 -> Breaker Load 12/1
  On/off Load 11/1 -> Breaker Load 11/1
  On/off Load 10/1 -> Breaker Load 10/1
  On/off Load 14/1 -> Breaker Load 14/1
  On/off Load 9/1 -> Breaker Load 9/1
  On/off Load 4/1 -> Breaker Load 4/1
  On/off Load 2/1 -> Breaker Load 2/1
  Ib_L2/1 -> [Ib_L2]
  Ia_L2/1 -> [Ia_L2]
  Ic_L2/1 -> [Ic_L2]
  Ic_L1/1 -> [Ic_L1]
  Ia_L1/1 -> [Ia_L1]
  Ib_L1/1 -> [Ib_L1]
  Ic_L6/1 -> [Ic_L6]
  Ia_L6/1 -> [Ia_L6]
  Ib_L6/1 -> [Ib_L6]
  Ic_L5/1 -> [Ic_L5]
  Ib_L5/1 -> [Ib_L5]
  Ia_L5/1 -> [Ia_L5]
  Ia_L4/1 -> [Ia_L4]
  Ib_L4/1 -> [Ib_L4]
  "  Ic_L4"/1 -> [Ic_L4]
  "  Ic_L3"/1 -> [Ic_L3]
  Ib_L3/1 -> [Ib_L3]
  Ia_L3/1 -> [Ia_L3]
  Ia_L7/1 -> [Ia_L7]
  Ib_L7/1 -> [Ib_L7]
  "  Ic_L7"/1 -> [Ic_L7]
  Ia_L8/1 -> [Ia_L8]
  Ib_L8/1 -> [Ib_L8]
  "  Ic_L8"/1 -> [Ic_L8]
  "  Ic_L9"/1 -> [Ic_L9]
  Ia_L9/1 -> [Ia_L9]
  Ib_L9/1 -> [Ib_L9]
  Ib_L10/1 -> [Ib_L10]
  Ia_L10/1 -> [Ia_L10]
  Ic_L10/1 -> [Ic_L10]
  "  Ic_L11"/1 -> [Ic_L11]
  Ib_L11/1 -> [Ib_L11]
  Ia_L11/1 -> [Ia_L11]
  Ic_L12/1 -> [Ic_L12]
  Ia_L12/1 -> [Ia_L12]
  Ib_L12/1 -> [Ib_L12]
  Ic_L14/1 -> [Ic_L14]
  Ia_L14/1 -> [Ia_L14]
  Ib_L14/1 -> [Ib_L14]
  Control measurement2/1("              Out1") -> [Means2]
  On/off grid bus DC1/1 -> Breaker bus DC1/1
  On/off grid bus DC2 OP_max / min1/1(on / off) -> Breaker bus DC2/1
  Current Measurement1/1 -> [I_BusDC]
  [Means2] -> Grid Bi-directional Converter 1.2 300 (DC) / 150 V (AC) P_nom 3kW/1(Means2)
  Control measurement/1("              Out1") -> [Means]
  [Means] -> Grid Bi-directional Converter 1.1 300 (DC) / 150 V (AC) P_nom 3kW/1(Means)
  "Bus_8      "/1("Means_Bus8      ") -> f1/1
  On/off grid G1/1 -> Breaker G1/1
  Resources/2(temp) -> "  PV Array 2"/2(Temp2)
  On/off 1/1 -> Breaker1/1, Breaker/1
  On/off 3/1 -> Breaker5/1, Breaker4/1
  On/off 4/1 -> Breaker7/1, Breaker6/1
  Resource1/2(Ir) -> "  PV Array 1 10.5 kW"/1(Irradiance)
  Resource1/1(Temp) -> "  PV Array 1 10.5 kW"/2(Temp2)
  On/off Load 3/1 -> Breaker Load 3/1
  OP_max / min/1(on / off) -> Breaker3/1, Breaker2/1
  connections:
  Ic_L2/RConn1 -- Bus1/RConn3 -- Ic_L1/RConn1
  Ib_L2/RConn1 -- Bus1/RConn2 -- Ib_L1/RConn1
  Ia_L2/RConn1 -- Ia_L1/RConn1 -- Bus1/RConn1
  Line1 150m/RConn1 -- TDC1 220 V / 150 V 15 kVA/LConn1 -- Bus2/LConn1
  Line1 150m/RConn2 -- TDC1 220 V / 150 V 15 kVA/LConn2 -- Bus2/LConn2
  Line1 150m/RConn3 -- TDC1 220 V / 150 V 15 kVA/LConn3 -- Bus2/LConn3
  Ia_L3/LConn1 -- Line2 200m/RConn1 -- Bus5/RConn1
  Ib_L3/LConn1 -- Line2 200m/RConn2 -- Bus5/RConn2
  "  Ic_L3"/LConn1 -- Line2 200m/RConn3 -- Bus5/RConn3
  Breaker Load 2/LConn2 -- Line4 400m/LConn2 -- Line6 400m/LConn2 -- TDC2 220 V / 150 V 15 kVA/LConn2 -- Bus2/RConn2 -- Line3 150m/LConn2
  TDC2 220 V / 150 V 15 kVA/LConn3 -- Line6 400m/LConn3 -- Line4 400m/LConn3 -- Bus2/RConn3 -- Line3 150m/LConn3 -- Breaker Load 2/LConn3
  Breaker Load 4/LConn1 -- Ia_L7/LConn1 -- Ia_L4/LConn1 -- Ia_L5/RConn1 -- Bus4/RConn1
  Breaker Load 4/LConn2 -- Ib_L7/LConn1 -- Ib_L4/LConn1 -- Ib_L5/RConn1 -- Bus4/RConn2
  Breaker Load 4/LConn3 -- "  Ic_L7"/LConn1 -- "  Ic_L4"/LConn1 -- Ic_L5/RConn1 -- Bus4/RConn3
  Transformer (T1) 13.8 kV / 220 V 1.5 MVA/RConn1 -- Line5 400m/LConn1 -- Bus5/LConn1
  Transformer (T1) 13.8 kV / 220 V 1.5 MVA/RConn2 -- Line5 400m/LConn2 -- Bus5/LConn2
  Transformer (T1) 13.8 kV / 220 V 1.5 MVA/RConn3 -- Line5 400m/LConn3 -- Bus5/LConn3
  Breaker Load 3/LConn1 -- Bus3/RConn1 -- Ia_L6/RConn1
  Breaker Load 3/LConn2 -- Bus3/RConn2 -- Ib_L6/RConn1
  Breaker Load 3/LConn3 -- Ic_L6/RConn1 -- Bus3/RConn3
  Transformer (T1) 13.8 kV / 220 V 1.5 MVA/LConn1 -- Line11 3km/LConn1 -- Bus6/LConn1
  Transformer (T1) 13.8 kV / 220 V 1.5 MVA/LConn2 -- Line11 3km/LConn2 -- Bus6/LConn2
  Bus6/LConn3 -- Line11 3km/LConn3 -- Transformer (T1) 13.8 kV / 220 V 1.5 MVA/LConn3
  Bus11/LConn1 -- Ia_L9/LConn1 -- Ia_L12/LConn1
  Ib_L9/LConn1 -- Ib_L12/LConn1 -- Bus11/LConn2
  "  Ic_L9"/LConn1 -- Ic_L12/LConn1 -- Bus11/LConn3
  Breaker MG/RConn1 -- Ia_L11/LConn1 -- Line13 3km/LConn1
  Breaker MG/RConn2 -- Line13 3km/LConn2 -- Ib_L11/LConn1
  Breaker MG/RConn3 -- Line13 3km/LConn3 -- "  Ic_L11"/LConn1
  Transformer (T2) 13.8 kV / 220 V 1.5 MVA/RConn1 -- Bus4/LConn1
  Transformer (T2) 13.8 kV / 220 V 1.5 MVA/RConn2 -- Bus4/LConn2
  Transformer (T2) 13.8 kV / 220 V 1.5 MVA/RConn3 -- Bus4/LConn3
  Breaker G1/RConn1 -- Bus7/LConn1 -- Transformer (T2) 13.8 kV / 220 V 1.5 MVA/LConn1
  Breaker G1/RConn2 -- Bus7/LConn2 -- Transformer (T2) 13.8 kV / 220 V 1.5 MVA/LConn2
  Breaker G1/RConn3 -- Bus7/LConn3 -- Transformer (T2) 13.8 kV / 220 V 1.5 MVA/LConn3
  Primary (69 kV)/LConn2 -- Main Grid 69 kV Inf/RConn2
  Transformer (T3) 69kV / 13.8 kV 4 MVA/RConn1 -- Secundario 13.8 kV LL/LConn1
  Primary (69 kV)/RConn3 -- Transformer (T3) 69kV / 13.8 kV 4 MVA/LConn3
  Primary (69 kV)/RConn1 -- Transformer (T3) 69kV / 13.8 kV 4 MVA/LConn1
  Transformer (T3) 69kV / 13.8 kV 4 MVA/RConn2 -- Secundario 13.8 kV LL/LConn2
  Primary (69 kV)/LConn1 -- Main Grid 69 kV Inf/RConn3
  Transformer (T3) 69kV / 13.8 kV 4 MVA/RConn3 -- Secundario 13.8 kV LL/LConn3
  Primary (69 kV)/LConn3 -- Main Grid 69 kV Inf/RConn1
  Primary (69 kV)/RConn2 -- Transformer (T3) 69kV / 13.8 kV 4 MVA/LConn2
  Load 14/LConn3 -- Bus14_1/RConn3 -- Bus14/LConn3
  Load 14/LConn2 -- Bus14_1/RConn2 -- Bus14/LConn2
  Load 14/LConn1 -- Bus14_1/RConn1 -- Bus14/LConn1
  Line3 150m/LConn1 -- Line4 400m/LConn1 -- Line6 400m/LConn1 -- TDC2 220 V / 150 V 15 kVA/LConn1 -- Bus2/RConn1 -- Breaker Load 2/LConn1
  Secundario 13.8 kV LL/RConn3 -- " Bus13"/LConn3
  Secundario 13.8 kV LL/RConn2 -- " Bus13"/LConn2
  Secundario 13.8 kV LL/RConn1 -- " Bus13"/LConn1
  Breaker PV/LConn3 -- TPV 13.8 KV / 250 V 1 MVA/LConn3
  TPV 13.8 KV / 250 V 1 MVA/LConn1 -- Breaker PV/LConn1
  TPV 13.8 KV / 250 V 1 MVA/LConn2 -- Breaker PV/LConn2
  TB 900 V / 220 V 55 kVA/LConn1 -- Grid Bi-directional converter AC /CD 2 Cascaded Topology/LConn1
  TB 900 V / 220 V 55 kVA/LConn2 -- Grid Bi-directional converter AC /CD 2 Cascaded Topology/LConn2
  TB 900 V / 220 V 55 kVA/LConn3 -- Grid Bi-directional converter AC /CD 2 Cascaded Topology/LConn3
  "Breaker BESS "/RConn1 -- Bus1/LConn1
  "Breaker BESS "/RConn2 -- Bus1/LConn2
  "Breaker BESS "/RConn3 -- Bus1/LConn3
  TB 900 V / 220 V 55 kVA/RConn2 -- "Breaker BESS "/LConn2
  TB 900 V / 220 V 55 kVA/RConn3 -- "Breaker BESS "/LConn3
  TB 900 V / 220 V 55 kVA/RConn1 -- "Breaker BESS "/LConn1
  " Bus13"/RConn3 -- Breaker MG/LConn3
  " Bus13"/RConn2 -- Breaker MG/LConn2
  " Bus13"/RConn1 -- Breaker MG/LConn1
  Unbalanced AC  Load 2/LConn1 -- Load 2/RConn1
  Unbalanced AC  Load 2/LConn2 -- Load 2/RConn2
  Unbalanced AC  Load 2/LConn3 -- Load 2/RConn3
  "Grid Inverter PV 480 / 250 DC / AC "/RConn1 -- TPV 13.8 KV / 250 V 1 MVA/RConn1
  "Grid Inverter PV 480 / 250 DC / AC "/RConn2 -- TPV 13.8 KV / 250 V 1 MVA/RConn2
  "Grid Inverter PV 480 / 250 DC / AC "/RConn3 -- TPV 13.8 KV / 250 V 1 MVA/RConn3
  "  PV Array 2"/LConn1 -- "Grid Inverter PV 480 / 250 DC / AC "/LConn1
  "  PV Array 2"/LConn2 -- "Grid Inverter PV 480 / 250 DC / AC "/LConn2
  "BESS 2 "/LConn1 -- Grid Bi-directional converter AC /CD 2 Cascaded Topology/RConn1
  "BESS 2 "/LConn2 -- Grid Bi-directional converter AC /CD 2 Cascaded Topology/RConn2
  "BESS 2 "/LConn3 -- Grid Bi-directional converter AC /CD 2 Cascaded Topology/RConn3
  "BESS 2 "/LConn4 -- Grid Bi-directional converter AC /CD 2 Cascaded Topology/RConn4
  "BESS 2 "/LConn5 -- Grid Bi-directional converter AC /CD 2 Cascaded Topology/RConn5
  "BESS 2 "/LConn6 -- Grid Bi-directional converter AC /CD 2 Cascaded Topology/RConn6
  Line13 3km/RConn1 -- Ia_L13/LConn1
  Line13 3km/RConn2 -- Ib_L13/LConn1
  Line13 3km/RConn3 -- Ic_L13/LConn1
  AC  Load 12/LConn1 -- Breaker Load 12/RConn1
  AC  Load 12/LConn2 -- Breaker Load 12/RConn2
  AC  Load 12/LConn3 -- Breaker Load 12/RConn3
  Breaker Load 11/LConn1 -- Bus11/RConn1
  Breaker Load 11/LConn2 -- Bus11/RConn2
  Breaker Load 11/LConn3 -- Bus11/RConn3
  AC  Load 11/LConn3 -- Breaker Load 11/RConn3
  AC  Load 11/LConn1 -- Breaker Load 11/RConn1
  AC  Load 11/LConn2 -- Breaker Load 11/RConn2
  Line12 6km/RConn1 -- Bus10/LConn1
  Line12 6km/RConn2 -- Bus10/LConn2
  Line12 6km/RConn3 -- Bus10/LConn3
  Breaker Load 10/LConn1 -- Bus10/RConn1
  Breaker Load 10/LConn2 -- Bus10/RConn2
  Breaker Load 10/LConn3 -- Bus10/RConn3
  AC  Load 10/LConn3 -- Breaker Load 10/RConn3
  AC  Load 10/LConn2 -- Breaker Load 10/RConn2
  AC  Load 10/LConn1 -- Breaker Load 10/RConn1
  AC  Load 14/LConn1 -- Breaker Load 14/RConn1
  AC  Load 14/LConn2 -- Breaker Load 14/RConn2
  AC  Load 14/LConn3 -- Breaker Load 14/RConn3
  AC  Load 4/LConn1 -- Breaker Load 4/RConn1
  AC  Load 4/LConn2 -- Breaker Load 4/RConn2
  AC  Load 4/LConn3 -- Breaker Load 4/RConn3
  Breaker Load 2/RConn1 -- Load 2/LConn1
  Breaker Load 2/RConn2 -- Load 2/LConn2
  Load 2/LConn3 -- Breaker Load 2/RConn3
  Line2 200m/LConn1 -- Ia_L2/LConn1
  Line2 200m/LConn2 -- Ib_L2/LConn1
  Line2 200m/LConn3 -- Ic_L2/LConn1
  Line1 150m/LConn1 -- Ia_L1/LConn1
  Line1 150m/LConn2 -- Ib_L1/LConn1
  Line1 150m/LConn3 -- Ic_L1/LConn1
  Line6 400m/RConn1 -- Ia_L6/LConn1
  Line6 400m/RConn2 -- Ib_L6/LConn1
  Line6 400m/RConn3 -- Ic_L6/LConn1
  Line5 400m/RConn1 -- Ia_L5/LConn1
  Line5 400m/RConn2 -- Ib_L5/LConn1
  Line5 400m/RConn3 -- Ic_L5/LConn1
  Line4 400m/RConn1 -- Ia_L4/RConn1
  Line4 400m/RConn2 -- Ib_L4/RConn1
  Line4 400m/RConn3 -- "  Ic_L4"/RConn1
  Line3 150m/RConn1 -- Ia_L3/RConn1
  Line3 150m/RConn2 -- Ib_L3/RConn1
  Line3 150m/RConn3 -- "  Ic_L3"/RConn1
  Line7 100m/RConn1 -- Ia_L7/RConn1
  Line7 100m/RConn3 -- "  Ic_L7"/RConn1
  Line7 100m/RConn2 -- Ib_L7/RConn1
  Line8 2km/RConn1 -- Ia_L8/RConn1
  Line8 2km/RConn2 -- Ib_L8/RConn1
  Line8 2km/RConn3 -- "  Ic_L8"/RConn1
  Line9 6km/RConn1 -- Ia_L9/RConn1
  Line9 6km/RConn3 -- "  Ic_L9"/RConn1
  Line9 6km/RConn2 -- Ib_L9/RConn1
  Line10 6km/RConn1 -- Ia_L10/LConn1
  Line10 6km/RConn2 -- Ib_L10/LConn1
  Line10 6km/RConn3 -- Ic_L10/LConn1
  Line11 3km/RConn3 -- "  Ic_L11"/RConn1
  Line11 3km/RConn2 -- Ib_L11/RConn1
  Line11 3km/RConn1 -- Ia_L11/RConn1
  Line12 6km/LConn1 -- Ia_L12/RConn1
  Line12 6km/LConn2 -- Ib_L12/RConn1
  Line12 6km/LConn3 -- Ic_L12/RConn1
  Line14 2km/RConn1 -- Ia_L14/RConn1
  Line14 2km/RConn2 -- Ib_L14/RConn1
  Line14 2km/RConn3 -- Ic_L14/RConn1
  Ia_L14/LConn1 -- Bus14/RConn1
  Ib_L14/LConn1 -- Bus14/RConn2
  Ic_L14/LConn1 -- Bus14/RConn3
  Bus12/RConn1 -- Breaker Load 12/LConn1
  Bus12/RConn2 -- Breaker Load 12/LConn2
  Breaker Load 12/LConn3 -- Bus12/RConn3
  Bus12/LConn3 -- Ic_L10/RConn1
  Bus12/LConn2 -- Ib_L10/RConn1
  Bus12/LConn1 -- Ia_L10/RConn1
  Breaker bus DC2/RConn3 -- TDC2 220 V / 150 V 15 kVA/RConn3 -- Control measurement2/LConn1
  Control measurement/LConn2 -- TDC1 220 V / 150 V 15 kVA/RConn2 -- Breaker bus DC1/RConn2
  Breaker bus DC2/RConn2 -- TDC2 220 V / 150 V 15 kVA/RConn2 -- Control measurement2/LConn2
  Control measurement/LConn3 -- TDC1 220 V / 150 V 15 kVA/RConn1 -- Breaker bus DC1/RConn1
  DC Load/RConn1 -- Breaker5/RConn1 -- Breaker1/LConn1 -- Breaker7/RConn1 -- Breaker3/LConn1
  Breaker bus DC2/RConn1 -- TDC2 220 V / 150 V 15 kVA/RConn1 -- Control measurement2/LConn3
  Breaker4/RConn1 -- DC Load/LConn1 -- Current Measurement1/LConn1 -- Breaker2/LConn1 -- Breaker6/RConn1
  Control measurement/LConn1 -- TDC1 220 V / 150 V 15 kVA/RConn3 -- Breaker bus DC1/RConn3
  Bus AC / DC 2/LConn3 -- Grid Bi-directional Converter 1.2 300 (DC) / 150 V (AC) P_nom 3kW/LConn3
  Bus AC / DC 2/LConn1 -- Grid Bi-directional Converter 1.2 300 (DC) / 150 V (AC) P_nom 3kW/LConn1
  Bus AC / DC 2/LConn2 -- Grid Bi-directional Converter 1.2 300 (DC) / 150 V (AC) P_nom 3kW/LConn2
  Bus AC / DC 1/RConn2 -- Breaker bus DC1/LConn2
  Bus AC / DC 2/RConn3 -- Breaker bus DC2/LConn3
  Bus AC / DC 1/LConn1 -- Grid Bi-directional Converter 1.1 300 (DC) / 150 V (AC) P_nom 3kW/LConn1
  Bus AC / DC 2/RConn1 -- Breaker bus DC2/LConn1
  Grid Bi-directional Converter 1.1 300 (DC) / 150 V (AC) P_nom 3kW/RConn1 -- Breaker/RConn1
  Bus AC / DC 1/LConn2 -- Grid Bi-directional Converter 1.1 300 (DC) / 150 V (AC) P_nom 3kW/LConn2
  Bus AC / DC 1/LConn3 -- Grid Bi-directional Converter 1.1 300 (DC) / 150 V (AC) P_nom 3kW/LConn3
  Bus AC / DC 1/RConn1 -- Breaker bus DC1/LConn1
  Bus AC / DC 2/RConn2 -- Breaker bus DC2/LConn2
  Bus AC / DC 1/RConn3 -- Breaker bus DC1/LConn3
  TG 13.8 kV / 2400 V 3.5 MVA/LConn1 -- Breaker G1/LConn1
  TG 13.8 kV / 2400 V 3.5 MVA/LConn3 -- Breaker G1/LConn3
  Diesel_ 3MVA/LConn1 -- Bus8/LConn1
  Bus8/RConn1 -- TG 13.8 kV / 2400 V 3.5 MVA/RConn1
  Diesel_ 3MVA/LConn2 -- Bus8/LConn2
  TG 13.8 kV / 2400 V 3.5 MVA/LConn2 -- Breaker G1/LConn2
  Diesel_ 3MVA/LConn3 -- Bus8/LConn3
  Bus8/RConn2 -- TG 13.8 kV / 2400 V 3.5 MVA/RConn2
  Bus8/RConn3 -- TG 13.8 kV / 2400 V 3.5 MVA/RConn3
  Boost -buck Bi-directional converter DC /CD 1 0.65 kW/LConn1 -- Battery Energy Storage System (BESS) 1/LConn1
  Boost -buck Bi-directional converter DC /CD 1 0.65 kW/LConn2 -- Battery Energy Storage System (BESS) 1/LConn2
  Current Measurement1/RConn1 -- Breaker/LConn1
  Grid Bi-directional Converter 1.1 300 (DC) / 150 V (AC) P_nom 3kW/RConn2 -- Breaker1/RConn1
  Grid Bi-directional Converter 1.2 300 (DC) / 150 V (AC) P_nom 3kW/RConn2 -- Breaker3/RConn1
  Grid Bi-directional Converter 1.2 300 (DC) / 150 V (AC) P_nom 3kW/RConn1 -- Breaker2/RConn1
  Boost -buck Bi-directional converter DC /CD 1 0.65 kW/RConn1 -- Breaker4/LConn1
  Breaker5/LConn1 -- Boost -buck Bi-directional converter DC /CD 1 0.65 kW/RConn2
  "Boost converter DC /CD 2 5 kHz - 300V "/LConn1 -- Breaker6/LConn1
  "Boost converter DC /CD 2 5 kHz - 300V "/LConn2 -- Breaker7/LConn1
  "  PV Array 1 10.5 kW"/LConn2 -- "Boost converter DC /CD 2 5 kHz - 300V "/RConn2
  "  PV Array 1 10.5 kW"/LConn1 -- "Boost converter DC /CD 2 5 kHz - 300V "/RConn1
  Line9 6km/LConn3 -- Bus6/RConn3 -- Line10 6km/LConn3 -- Bus AC PV/RConn3
  Line9 6km/LConn2 -- Bus6/RConn2 -- Bus AC PV/RConn2 -- Line10 6km/LConn2
  Line9 6km/LConn1 -- Bus6/RConn1 -- Bus AC PV/RConn1 -- Line10 6km/LConn1
  Bus AC PV/LConn1 -- Breaker PV/RConn1
  Bus AC PV/LConn2 -- Breaker PV/RConn2
  Bus AC PV/LConn3 -- Breaker PV/RConn3
  Load 3/LConn3 -- Breaker Load 3/RConn3
  Load 3/LConn1 -- Breaker Load 3/RConn1
  Unbalanced AC  Load 3/LConn3 -- Load 3/RConn3
  Unbalanced AC  Load 3/LConn1 -- Load 3/RConn1
  Load 3/LConn2 -- Breaker Load 3/RConn2
  Unbalanced AC  Load 3/LConn2 -- Load 3/RConn2
  Non Linear AC  Load 9/LConn1 -- Breaker Load 9/RConn1
  Non Linear AC  Load 9/LConn2 -- Breaker Load 9/RConn2
  Non Linear AC  Load 9/LConn3 -- Breaker Load 9/RConn3
  Line14 2km/LConn1 -- Bus9/LConn1 -- Ia_L8/LConn1
  Line14 2km/LConn2 -- Bus9/LConn2 -- Ib_L8/LConn1
  Line14 2km/LConn3 -- Bus9/LConn3 -- "  Ic_L8"/LConn1
  Bus9/RConn3 -- Breaker Load 9/LConn3
  Bus9/RConn2 -- Breaker Load 9/LConn2
  Breaker Load 9/LConn1 -- Bus9/RConn1
  Bus3/LConn2 -- Line7 100m/LConn2
  Bus3/LConn3 -- Line7 100m/LConn3
  Bus3/LConn1 -- Line7 100m/LConn1
  Bus7/RConn1 -- Line8 2km/LConn1
  Bus7/RConn2 -- Line8 2km/LConn2
  Bus7/RConn3 -- Line8 2km/LConn3
  Load 14/RConn1 -- Breaker Load 14/LConn1
  Load 14/RConn2 -- Breaker Load 14/LConn2
  Load 14/RConn3 -- Breaker Load 14/LConn3
  Bus14_1/LConn1 -- Ia_L13/RConn1
  Bus14_1/LConn2 -- Ib_L13/RConn1
  Bus14_1/LConn3 -- Ic_L13/RConn1

== system Model_14Bus_AC_DC_Microgrid/  PV Array 1 10.5 kW ==
  note: DC Bus
  note: 10.5 - kW  PV Array
      | 42 * SunTech STP - 250S-20 /Wd  (Nser=6 Npar=7)
  Irradiance : Inport
  Temp2 : Inport  Port=2
  PV Array : spsPVArrayLib/PV Array  Npar=7  Nser=6  PlotType=array @ 1000 W/m2 & specified temperatures  S_vec="[ 1000  250 ]"  Temp_C_vec="[0 25 50  ]"  ModuleName=User-defined  PlotWhenSelected=off  Pm=250.205  Ncell=96  Voc=37.4  Isc=8.63  Vm=30.7  Im=8.15  beta_Voc_pc=-0.34  alpha_Isc_pc=0.050  beta_Voc=-0.12716  alpha_Isc=0.004315  IL=8.6686  I0=1.3965e-10  nI=0.6105  Rsh=311.9016  Rs=0.26776  RobustModel=off  RobustCellTemperature=313.3991  BAL=on  Tc=Tc  Tfilter=5e-5
  + : PMIOPort  Tag=PMCPort  Side=Left
  - : PMIOPort  Tag=PMCPort  Port=2  Side=Left
  tag scope: m_PV=global
  wires:
  Temp2/1 -> PV Array/2
  Irradiance/1 -> PV Array/1
  PV Array/1 -> [m_PV]
  connections:
  PV Array/RConn1 -- +/RConn1
  PV Array/RConn2 -- -/RConn1

== system Model_14Bus_AC_DC_Microgrid/  PV Array 2 ==
  note: DC Bus
  Irradiance : Inport
  Temp2 : Inport  Port=2
  PV Array : spsPVArrayLib/PV Array  Npar=250  Nser=7  PlotType=array @ 1000 W/m2 & specified temperatures  S_vec="[ 1000  500  100 ]"  Temp_C_vec="[ 45 25  ]"  ModuleName=SunPower SPR-415E-WHT-D  PlotWhenSelected=off  Pm=414.801  Ncell=128  Voc=85.3  Isc=6.09  Vm=72.9  Im=5.69  beta_Voc_pc=-0.229  alpha_Isc_pc=0.030706  beta_Voc=-0.19534  alpha_Isc=0.00187  IL=6.0978  I0=7.1698e-13  nI=0.87223  Rsh=419.7781  Rs=0.53711  RobustModel=off  RobustCellTemperature=313.3991  BAL=on  Tc=1e-6  Tfilter=5e-5
      settings: AttributesFormatString=|
      | %<ModuleName>
      | %<Nser>-module string
      | %<Npar> parallel strings
  + : PMIOPort  Tag=PMCPort  Side=Left
  - : PMIOPort  Tag=PMCPort  Port=2  Side=Left
  tag scope: meas_PV=global
  wires:
  PV Array/1 -> [meas_PV]
  Irradiance/1 -> PV Array/1
  Temp2/1 -> PV Array/2
  connections:
  PV Array/RConn2 -- -/RConn1
  +/RConn1 -- PV Array/RConn1

== system Model_14Bus_AC_DC_Microgrid/BESS 2  ==
  Battery : spsBatteryLib/Battery  BatType=Nickel-Metal-Hydride  NomV=650  NomQ=1.5  SOC=80  Batt_Tr=30  PresetModel=on  MaxQ=1.6154  MinV=487.5  FullV=765.678  Dis_rate=0.3  R=4.3333  Normal_OP=1.4423  expZone="[705.0847           0.3]"
      settings: LibrarySourceBlock=electricdrivelib/Extra Sources/Battery
  Battery1 : spsBatteryLib/Battery  BatType=Nickel-Metal-Hydride  NomV=650  NomQ=1.5  SOC=80  Batt_Tr=30  PresetModel=on  MaxQ=1.6154  MinV=487.5  FullV=765.678  Dis_rate=0.3  R=4.3333  Normal_OP=1.4423  expZone="[705.0847           0.3]"
      settings: LibrarySourceBlock=electricdrivelib/Extra Sources/Battery
  Battery2 : spsBatteryLib/Battery  BatType=Nickel-Metal-Hydride  NomV=650  NomQ=1.5  SOC=80  Batt_Tr=30  PresetModel=on  MaxQ=1.6154  MinV=487.5  FullV=765.678  Dis_rate=0.3  R=4.3333  Normal_OP=1.4423  expZone="[705.0847           0.3]"
      settings: LibrarySourceBlock=electricdrivelib/Extra Sources/Battery
  + B1 : PMIOPort  Side=Left
  - B1 : PMIOPort  Port=2  Side=Left
  + B2 : PMIOPort  Port=3  Side=Left
  - B2 : PMIOPort  Port=4  Side=Left
  + B3 : PMIOPort  Port=5  Side=Left
  - B3 : PMIOPort  Port=6  Side=Left
  connections:
  Battery2/LConn1 -- + B3/RConn1
  Battery/LConn1 -- + B1/RConn1
  Battery1/LConn1 -- + B2/RConn1
  Battery2/LConn2 -- - B3/RConn1
  Battery1/LConn2 -- - B2/RConn1
  Battery/LConn2 -- - B1/RConn1
